simulink subsystem "SiEngineCoreNA"  (R2023b)
settings: Solver=VariableStepAuto  StartTime=0.0  StopTime=10.0  RelTol=1e-3
undefined symbols (not defined in the file): EnvAbsPrs, EnvAirTemp, EnvCpAir, EnvRair, PlntEngCEng, PlntEngCpExh, PlntEngEgrArea, PlntEngExhSysVol, PlntEngGasLhv, PlntEngRexh, PlntEngTauCool, PlntEngTCoolInit, PlntEngTCoolMax, PlntEngTCoolStart, PlntEngThrAngToC, PlntEngVexh, ThrAngToC
libraries: autolibfundflw x10, autolibfundflwcommon x2, simulink x1, autolibpowerinfoutils x1, autolibcoreeng x1
settings Model: ModifiedByFormat=The MathWorks, Inc.  Creator=The MathWorks, Inc.  LastModifiedBy=The MathWorks, Inc.
settings SolverCC: MaxZcPerStep=1
settings OptimizationCC: ReuseModelBlockBuffer=off
settings DebuggingCC: UnconnectedInputMsg=warning  UnconnectedOutputMsg=warning  UnconnectedLineMsg=warning
settings ModelReferenceCC: EnableRefExpFcnMdlSchedulingChecks=on
settings RTWCC: DLArmComputeVersion=19.05

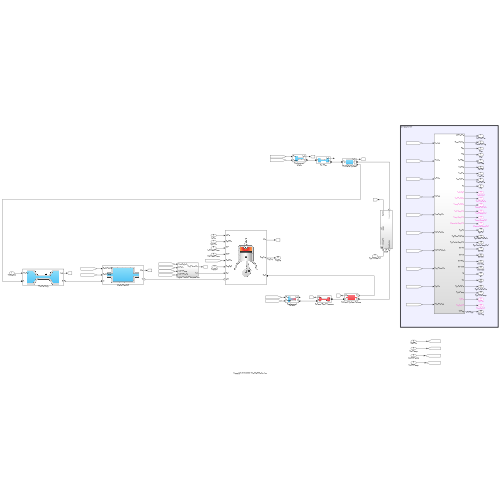
[thumbnail: Simulink's stored preview of the top-level diagram]
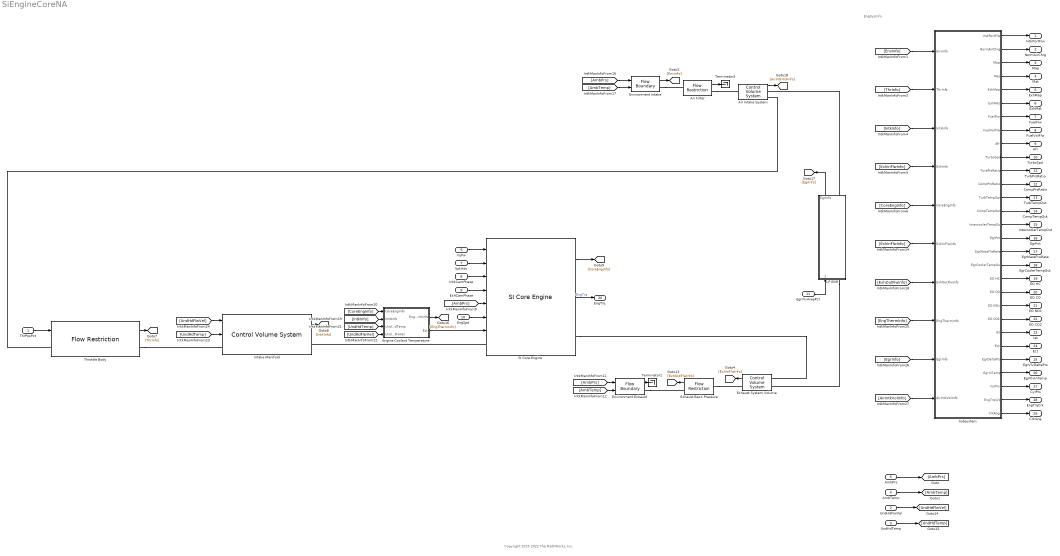
== system SiEngineCoreNA ==
  note: EngSysInfo
  note: Copyright 2015-2022 The MathWorks, Inc.
  ThrPosPct : Inport
  UndHdFlwVel : Inport  Port=2
  UndHdTemp : Inport  Port=3
  AmbTemp : Inport  Port=4
  AmbPrs : Inport  Port=5
  InjPw : Inport  Port=6
  SpkAdv : Inport  Port=7
  IntkCamPhase : Inport  Port=8
  ExhCamPhase : Inport  Port=9
  EngSpd : Inport  Port=10
  EgrVlvAreaPct : Inport  Port=11
  Air Filter : autolibfundflw/Flow Restriction  AreaPopup=Constant  ImageTypePopup=Cold  gamma=EnvCpAir/(EnvCpAir-EnvRair)  R=EnvRair  Plim=0.99  Aorf_cnst=PlntEngAFArea  Cd_cnst=1  Cd_ext=1  Dthr=50  ThrCd=[0.001; 0.735]  ThrAngBpts=[0; 90]
  Air Intake System : autolibfundflw/Control Volume System  NumInletPorts=1  NumOutletPorts=2  HeatTransferModelPopup=Constant  ImageTypePopup=Cold  Vch=PlntEngIntkVol  Pinit=EnvAbsPrs  Tinit=EnvAirTemp  R=EnvRair  cp=EnvCpAir  q_he=0  ext_tbl=[40 160 740 2000]  ext_bpts=linspace(0,180,4)  Aext_conv=0.125  m_wall=7  cp_wall=900  Tmass=293.15  Dext_cond=0.004  Aext_cond=0.003  kext=25  Dint_cond=0.004  Aint_cond=0.003  kint=25  int_tbl=[40 160 740 2000]  int_bpts=linspace(0.0020,0.1100,4)  Aint_conv=0.125
  Engine Coolant Temperature : Subsystem
  Environment Exhaust : autolibfundflw/Flow Boundary  PrsTempSrcPopup=External input  ImageTypePopup=Hot  Pcnst=101325  Tcnst=298.15  cp=EnvCpAir
  Environment Intake : autolibfundflw/Flow Boundary  PrsTempSrcPopup=External input  ImageTypePopup=Cold  Pcnst=101325  Tcnst=298.15  cp=EnvCpAir
  Exhaust Back Pressure : autolibfundflw/Flow Restriction  AreaPopup=Constant  ImageTypePopup=Hot  gamma=PlntEngCpExh/(PlntEngCpExh-PlntEngRexh)  R=PlntEngRexh  Plim=0.99  Aorf_cnst=PlntEngExhSysArea  Cd_cnst=1  Cd_ext=1  Dthr=50  ThrCd=[0.001; 0.735]  ThrAngBpts=[0; 90]
  Exhaust System Volume : autolibfundflw/Control Volume System  NumInletPorts=2  NumOutletPorts=1  HeatTransferModelPopup=Constant  ImageTypePopup=Hot  Vch=PlntEngExhSysVol+PlntEngVexh  Pinit=101325  Tinit=298  R=PlntEngRexh  cp=PlntEngCpExh  q_he=0  ext_tbl=[40 160 740 2000]  ext_bpts=linspace(0,180,4)  Aext_conv=0.125  m_wall=7  cp_wall=900  Tmass=293.15  Dext_cond=0.004  Aext_cond=0.003  kext=25  Dint_cond=0.004  Aint_cond=0.003  kint=25  int_tbl=[40 160 740 2000]  int_bpts=linspace(0.0020,0.1100,4)  Aint_conv=0.125
  Intake Manifold : autolibfundflw/Control Volume System  NumInletPorts=1  NumOutletPorts=1  HeatTransferModelPopup=External wall convection  ImageTypePopup=Cold  Vch=PlntEngVint  Pinit=101325  Tinit=298  R=EnvRair  cp=EnvCpAir  q_he=0  ext_tbl=[40 160 740 2000]  ext_bpts=linspace(0,180,4)  Aext_conv=0.125  m_wall=7  cp_wall=900  Tmass=293.15  Dext_cond=0.004  Aext_cond=0.003  kext=25  Dint_cond=0.004  Aint_cond=0.003  kint=25  int_tbl=[40 160 740 2000]  int_bpts=linspace(0.0020,0.1100,4)  Aint_conv=0.125
  LP EGR : Subsystem  Variant=on  VariantControlMode=label  VariantControl=Choice  LabelModeActiveChoice=LpEGR
  SI Core Engine : autolibcoreeng/SI Core Engine  AirMassFlowOptionPopup=Dual-Independent Variable Cam Phasing  TrqOptionPopup=Torque Structure  NCyl=PlntEngNCyl  Cps=PlntEngCps  Vd=PlntEngVd  Rair=EnvRair  Pstd=EnvAbsPrs  Tstd=EnvAirTemp  f_nv=PlntEngNv  f_nv_prs_bpt=PlntEngNvPrBpt  f_nv_n_bpt=PlntEngNvSpdBpt  f_vivc=PlntEngVivc  f_vivc_icp_bpt=PlntEngVivcBpt  f_tm_corr=PlntEngTmCorr  f_tm_corr_nd_bpt=PlntEngTmCorrNdBpt  f_tm_corr_n_bpt=PlntEngTmCorrNBpt  f_mdot_intk=PlntEngNAMdotIntk  f_mdot_intk_ecp_bpt=PlntEngMdotIntkEcpBpt  f_mdot_trpd_bpt=PlntEngMdotTrpdBpt  f_mdot_air_corr=PlntEngMdotAirCorr  f_mdot_air_corr_ld_bpt=PlntEngMdotAirCorrLdBpt  f_mdot_air_n_bpt=PlntEngMdotAirCorrNBpt  EnableCrkSignalsCheckbox=off  f_crk_firing_frac_bpt=[-1 0 1]  f_crk_prs=PlntEngCrkPrs  f_crk_btq=PlntEngCrkBtq  f_crk_n_bpt=PlntEngCrkNBpt  f_crk_l_bpt=PlntEngCrkLBpt  f_crk_ang_bpt=PlntEngCrkAngBpt  f_crk_tdc_ang=PlntEngCrkTdcAng  f_tq_nl=PlntEngTqTbl  f_tq_nl_l_bpt=PlntEngTqTblLBpt  f_tq_nl_n_bpt=PlntEngTqTblNBpt  f_tq_inr=PlntEngInTrqMapNA  f_tq_fric=PlntEngTqFricNA  f_fric_temp_mod=PlntEngFricTMod  f_fric_temp_bpt=PlntEngFricTBpt  f_tq_pump=PlntEngTqPumpNA  f_sa_opt=PlntEngSAOptNA  f_tq_inr_l_bpt=PlntEngInTrqLdBptNA  f_tq_inr_n_bpt=PlntEngInTrqSpdBptNA  f_m_sa=PlntEngMSa  f_del_sa_bpt=PlntEngDelSaBpt  f_m_lam=PlntEngMLam  f_m_lam_bpt=PlntEngMLamBpt  f_t_exh=PlntEngTexh  f_t_exh_l_bpt=PlntEngTexhLBpt  f_t_exh_n_bpt=PlntEngTexhNBpt  cp_exh=PlntEngCpExh  CO2EmissionsCheckbox=on  COEmissionsCheckbox=on  NOxEmissionsCheckbox=on  HCEmissionsCheckbox=on  PMEmissionsCheckbox=off  f_CO2_frac=PlntEngCO2Frac  f_CO_frac=PlntEngCOFrac  f_HC_frac=PlntEngHCFrac  f_NOx_frac=PlntEngNOxFrac  f_PM_frac=[0 0 0 0 0 0 0 0 0 0 0 0 0 0 0;0 0 0 0 0 0 0 0 0 0 0 0 0 0 0;0 0 0 0 0 0 0 0 0 0 0 0 0 0 0;0 0 0 0 0 0 0 0 0 0 0 0 0 0 0;0 0 0 0 0 0 0 0 0 0 0 0 0 0 0;0 0 0 0 0 0 0 0 0 0 0 0 0 0 0;0 0 0 0 0 0 0 0 0 0 0 0 0 0 0;0 0 0 0 0 0 0 0 0 0 0 0 0 0 0;0 0 0 0 0 0 0 0 0 0 0 0 0 0 0;0 0 0 0 0 0 0 0 0 0 0 0 0 0 0;0 0 0 0 0 0 0 0 0 0 0 0 0 0 0;0 0 0 0 0 0 0 0 0 0 0 0 0 0 0;0 0 0 0 0 0 0 0 0 0 0 0 0 0 0;0 0 0 0 0 0 0 0 0 0 0 0 0 0 0;0 0 0 0 0 0 0 0 0 0 0 0 0 0 0;0 0 0 0 0 0 0 0 0 0 0 0 0 0 0]  f_exhfrac_n_bpt=PlntEngExhFracNBpt  f_exhfrac_trq_bpt=PlntEngExhFracTqBpt  Sinj=PlntEngSinj  afr_stoich=PlntEngAfrStoich  fuel_lhv=PlntEngGasLhv  fuel_sg=PlntEngGasSg
  Subsystem : Subsystem
  Terminator1 : Terminator
  Terminator5 : Terminator
  Throttle Body : autolibfundflw/Flow Restriction  AreaPopup=Throttle body geometry  ImageTypePopup=Cold  gamma=EnvCpAir / (EnvCpAir - EnvRair)  R=EnvRair  Plim=0.99  Aorf_cnst=.1  Cd_cnst=1  Cd_ext=1  Dthr=PlntEngThrDia  ThrCd=PlntEngThrAngToC(:,2)  ThrAngBpts=PlntEngThrAngToC(:,1)
  IntkPortFlw : Outport  VectorParamsAs1DForOutWhenUnconnected=off
  NormAirChrg : Outport  Port=2  VectorParamsAs1DForOutWhenUnconnected=off
  Map : Outport  Port=3  VectorParamsAs1DForOutWhenUnconnected=off
  Mat : Outport  Port=4  VectorParamsAs1DForOutWhenUnconnected=off
  ExhMap : Outport  Port=5  VectorParamsAs1DForOutWhenUnconnected=off
  ExhMat : Outport  Port=6  VectorParamsAs1DForOutWhenUnconnected=off
  FuelFlw : Outport  Port=7  VectorParamsAs1DForOutWhenUnconnected=off
  FuelVolFlw : Outport  Port=8  VectorParamsAs1DForOutWhenUnconnected=off
  Afr : Outport  Port=9  VectorParamsAs1DForOutWhenUnconnected=off
  TurboSpd : Outport  Port=10  VectorParamsAs1DForOutWhenUnconnected=off
  TurbPrsRatio : Outport  Port=11  VectorParamsAs1DForOutWhenUnconnected=off
  CompPrsRatio : Outport  Port=12  VectorParamsAs1DForOutWhenUnconnected=off
  TurbTempOut : Outport  Port=13  VectorParamsAs1DForOutWhenUnconnected=off
  CompTempOut : Outport  Port=14  VectorParamsAs1DForOutWhenUnconnected=off
  IntercoolerTempOut : Outport  Port=15  VectorParamsAs1DForOutWhenUnconnected=off
  EgrPct : Outport  Port=16  VectorParamsAs1DForOutWhenUnconnected=off
  EgrMassFlwRate : Outport  Port=17  VectorParamsAs1DForOutWhenUnconnected=off
  EgrCoolerTempOut : Outport  Port=18  VectorParamsAs1DForOutWhenUnconnected=off
  EO HC : Outport  Port=19  VectorParamsAs1DForOutWhenUnconnected=off
  EO CO : Outport  Port=20  VectorParamsAs1DForOutWhenUnconnected=off
  EO NOx : Outport  Port=21  VectorParamsAs1DForOutWhenUnconnected=off
  EO CO2 : Outport  Port=22  VectorParamsAs1DForOutWhenUnconnected=off
  Iat : Outport  Port=23  VectorParamsAs1DForOutWhenUnconnected=off
  Ect : Outport  Port=24  VectorParamsAs1DForOutWhenUnconnected=off
  EgrVlvDeltaPrs : Outport  Port=25  VectorParamsAs1DForOutWhenUnconnected=off
  EgrVlvInTemp : Outport  Port=26  VectorParamsAs1DForOutWhenUnconnected=off
  CylPrs : Outport  Port=27  VectorParamsAs1DForOutWhenUnconnected=off
  EngTrqCrk : Outport  Port=28  VectorParamsAs1DForOutWhenUnconnected=off
  CrkAng : Outport  Port=29  VectorParamsAs1DForOutWhenUnconnected=off
  EngTrq : Outport  Port=30  VectorParamsAs1DForOutWhenUnconnected=off
  wires:
  [ExhInFlwInfo] -> Subsystem/4(ExhInfo)
  Subsystem/14(CompTempOut) -> CompTempOut/1
  Subsystem/29(CrkAng) -> CrkAng/1
  Subsystem/28(EngTrqCrk) -> EngTrqCrk/1
  Subsystem/12(CompPrsRatio) -> CompPrsRatio/1
  Subsystem/6(ExhMat) -> ExhMat/1
  Subsystem/8(FuelVolFlw) -> FuelVolFlw/1
  AmbTemp/1 -> [AmbTemp]
  Subsystem/13(TurbTempOut) -> TurbTempOut/1
  Subsystem/27(CylPrs) -> CylPrs/1
  Subsystem/15(IntercoolerTempOut) -> IntercoolerTempOut/1
  [UndHdFlwVel] -> Intake Manifold/1
  Subsystem/24(Ect) -> Ect/1
  Subsystem/11(TurbPrsRatio) -> TurbPrsRatio/1
  Subsystem/23(Iat) -> Iat/1
  Subsystem/10(TurboSpd) -> TurboSpd/1
  AmbPrs/1 -> [AmbPrs]
  Subsystem/22(EO CO2) -> EO CO2/1
  Subsystem/3(Map) -> Map/1
  Subsystem/9(Afr) -> Afr/1
  Subsystem/25(EgrDeltaPrs) -> EgrVlvDeltaPrs/1
  Subsystem/26(EgrInTemp) -> EgrVlvInTemp/1
  Subsystem/21(EO NOx) -> EO NOx/1
  Subsystem/4(Mat) -> Mat/1
  Subsystem/5(ExhMap) -> ExhMap/1
  [AirIntkVolInfo] -> Subsystem/10(AirIntkVolInfo)
  [AmbPrs] -> Environment Intake/1
  Subsystem/16(EgrPct) -> EgrPct/1
  [CoreEngInfo] -> Subsystem/5(CoreEngInfo)
  Subsystem/20(EO CO) -> EO CO/1
  Subsystem/7(FuelFlw) -> FuelFlw/1
  [EgrInfo] -> Subsystem/9(EgrInfo)
  [ExhOutFlwInfo] -> Subsystem/7(ExhOutFlwInfo)
  [EngThermInfo] -> Subsystem/8(EngThermInfo)
  [ExhInFlwInfo] -> Subsystem/6(ExhInFlwInfo)
  ThrPosPct/1 -> Throttle Body/1
  [UndHdTemp] -> Intake Manifold/2
  UndHdFlwVel/1 -> [UndHdFlwVel]
  UndHdTemp/1 -> [UndHdTemp]
  Intake Manifold/1 -> [IntkInfo]
  Exhaust Back Pressure/1 -> [ExhOutFlwInfo]
  [EnvInfo] -> Subsystem/1(EnvInfo)
  Environment Intake/1 -> [EnvInfo]
  Subsystem/18(EgrCoolerTempOut) -> EgrCoolerTempOut/1
  Exhaust System Volume/1 -> [ExhInFlwInfo]
  Environment Exhaust/1 -> Terminator1/1
  Subsystem/19(EO HC) -> EO HC/1
  [AmbTemp] -> Environment Exhaust/2
  Subsystem/2(NormAirChrg) -> NormAirChrg/1
  Subsystem/1(IntkPortFlw) -> IntkPortFlw/1
  [AmbPrs] -> Environment Exhaust/1
  [AmbTemp] -> Environment Intake/2
  Air Filter/1 -> Terminator5/1
  Throttle Body/1 -> [ThrInfo]
  [IntkInfo] -> Subsystem/3(IntkInfo)
  Subsystem/17(EgrMassFlwRate) -> EgrMassFlwRate/1
  Air Intake System/1 -> [AirIntkVolInfo]
  [ThrInfo] -> Subsystem/2(ThrInfo)
  SpkAdv/1 -> SI Core Engine/2
  ExhCamPhase/1 -> SI Core Engine/4
  IntkCamPhase/1 -> SI Core Engine/3
  EngSpd/1 -> SI Core Engine/6
  SI Core Engine/1 -> [CoreEngInfo]
  InjPw/1 -> SI Core Engine/1
  [UndHdTemp] -> Engine Coolant Temperature/3(UndHdTemp)
  Engine Coolant Temperature/2(Ect) -> SI Core Engine/7
  [IntkInfo] -> Engine Coolant Temperature/2(IntkInfo)
  [CoreEngInfo] -> Engine Coolant Temperature/1(CoreEngInfo)
  [AmbPrs] -> SI Core Engine/5
  [UndHdFlwVel] -> Engine Coolant Temperature/4(UndHdFlwVel)
  SI Core Engine/2 -> EngTrq/1  "EngTrq"
  Engine Coolant Temperature/1(EngThermInfo) -> [EngThermInfo]
  LP EGR/1(EgrInfo) -> [EgrInfo]
  EgrVlvAreaPct/1 -> LP EGR/1(EgrVlvAreaPct)
  connections:
  Throttle Body/LConn1 -- Air Intake System/RConn2
  Air Filter/RConn1 -- Air Intake System/LConn1
  Throttle Body/RConn1 -- Intake Manifold/LConn1
  Environment Intake/RConn1 -- Air Filter/LConn1
  Exhaust Back Pressure/LConn1 -- Exhaust System Volume/RConn1
  Environment Exhaust/RConn1 -- Exhaust Back Pressure/RConn1
  SI Core Engine/RConn1 -- Exhaust System Volume/LConn1
  SI Core Engine/LConn1 -- Intake Manifold/RConn1
  LP EGR/RConn1 -- Air Intake System/RConn1
  LP EGR/LConn1 -- Exhaust System Volume/LConn2

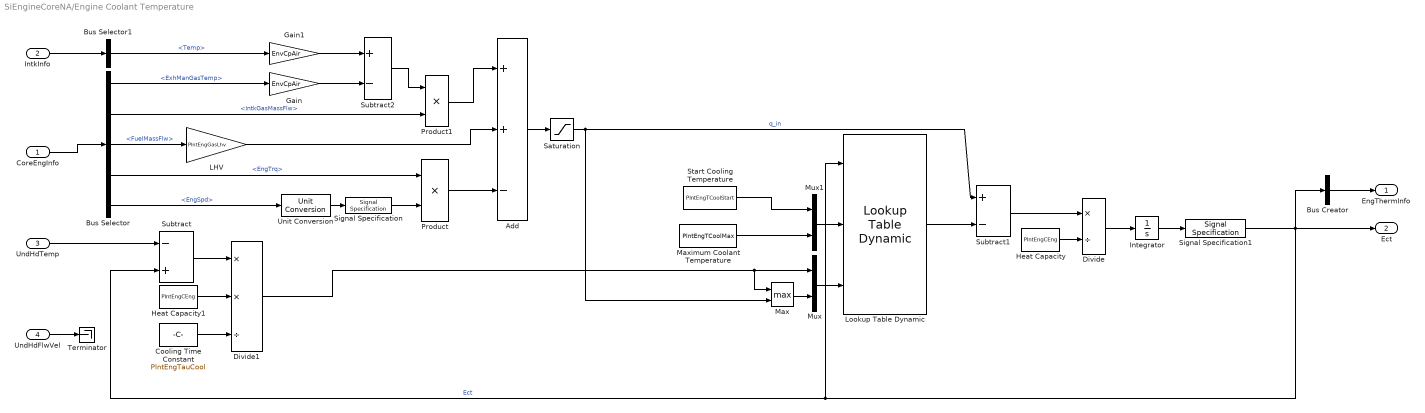
== system SiEngineCoreNA/Engine Coolant Temperature ==
  CoreEngInfo : Inport
  IntkInfo : Inport  Port=2
  UndHdTemp : Inport  Port=3
  UndHdFlwVel : Inport  Port=4
  Add : Sum  Inputs=++-
  Bus Creator : BusCreator  Inputs=1
  Bus Selector : BusSelector  OutputSignals=ExhManGasTemp,IntkGasMassFlw,FuelMassFlw,EngTrq,EngSpd
  Bus Selector1 : BusSelector  OutputSignals=Vol.Temp
  Cooling Time Constant : Constant  Value=PlntEngTauCool
  Divide : Product  Inputs=*/
  Divide1 : Product  Inputs=**/
  Gain : Gain  Gain=EnvCpAir
  Gain1 : Gain  Gain=EnvCpAir
  Heat Capacity : Constant  Value=PlntEngCEng
  Heat Capacity1 : Constant  Value=PlntEngCEng
  Integrator : Integrator  InitialCondition=PlntEngTCoolInit  LimitOutput=on  UpperSaturationLimit=PlntEngTCoolMax  LowerSaturationLimit=0  ZeroCross=off
  LHV : Gain  Gain=PlntEngGasLhv
  Lookup Table Dynamic : simulink/Lookup Tables/Lookup Table Dynamic  LookUpMeth=Interpolation-Use End Values  OutDataType=fixdt('double')  OutScaling=[]  OutputDataTypeScalingMode=Specify via dialog  OutDataTypeStr=double  DoSatur=off
  Max : MinMax  Function=max  Inputs=2  ZeroCross=off
  Maximum Coolant Temperature : Constant  Value=PlntEngTCoolMax
  Mux : Mux  Inputs=2
  Mux1 : Mux  Inputs=2
  Product : Product
  Product1 : Product
  Saturation : Saturate  UpperLimit=Inf  LowerLimit=0
  Signal Specification : SignalSpecification  Unit=rad/s
  Signal Specification1 : SignalSpecification  Unit=K
  Start Cooling Temperature : Constant  Value=PlntEngTCoolStart
  Subtract : Sum  Inputs=-+
  Subtract1 : Sum  Inputs=+-
  Subtract2 : Sum  Inputs=+-
  Terminator : Terminator
  Unit Conversion : UnitConversion
  EngThermInfo : Outport  Unit=K  VectorParamsAs1DForOutWhenUnconnected=off
  Ect : Outport  Port=2  Unit=K  VectorParamsAs1DForOutWhenUnconnected=off
  wires:
  Add/1 -> Saturation/1
  Product1/1 -> Add/1
  Bus Selector/2 -> Product1/2  "<IntkGasMassFlw>"
  Subtract2/1 -> Product1/1
  Integrator/1 -> Signal Specification1/1
  IntkInfo/1 -> Bus Selector1/1
  Bus Creator/1 -> EngThermInfo/1
  Max/1 -> Mux/2
  Lookup Table Dynamic/1 -> Subtract1/2
  Subtract1/1 -> Divide/1
  Divide/1 -> Integrator/1
  Bus Selector1/1 -> Gain1/1  "<Temp>"
  Gain1/1 -> Subtract2/1
  Bus Selector/1 -> Gain/1  "<ExhManGasTemp>"
  Bus Selector/3 -> LHV/1  "<FuelMassFlw>"
  CoreEngInfo/1 -> Bus Selector/1
  Cooling Time Constant/1 -> Divide1/3
  Bus Selector/5 -> Unit Conversion/1  "<EngSpd>"
  Product/1 -> Add/3
  LHV/1 -> Add/2
  Signal Specification/1 -> Product/2
  Saturation/1 -> Subtract1/1, Max/2  "q_in"
  Subtract/1 -> Divide1/1
  Start Cooling Temperature/1 -> Mux1/1
  Mux/1 -> Lookup Table Dynamic/3
  Heat Capacity1/1 -> Divide1/2
  Divide1/1 -> Mux/1, Max/1
  Mux1/1 -> Lookup Table Dynamic/2
  Bus Selector/4 -> Product/1  "<EngTrq>"
  Gain/1 -> Subtract2/2
  UndHdFlwVel/1 -> Terminator/1
  Signal Specification1/1 -> Ect/1, Bus Creator/1, Lookup Table Dynamic/1, Subtract/2  "Ect"
  Maximum Coolant Temperature/1 -> Mux1/2
  Unit Conversion/1 -> Signal Specification/1
  Heat Capacity/1 -> Divide/2
  UndHdTemp/1 -> Subtract/1

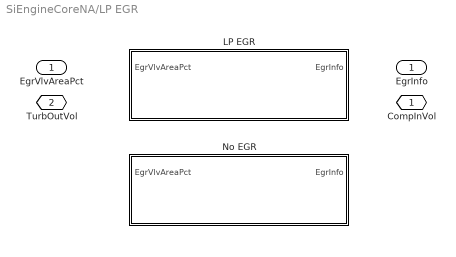
== system SiEngineCoreNA/LP EGR ==
  EgrVlvAreaPct : Inport
  LP EGR : Subsystem  VariantControl=LpEGR
  No EGR : Subsystem  VariantControl=NoEGR
  CompInVol : PMIOPort  Side=Right
  TurbOutVol : PMIOPort  Port=2  Side=Left
  EgrInfo : Outport

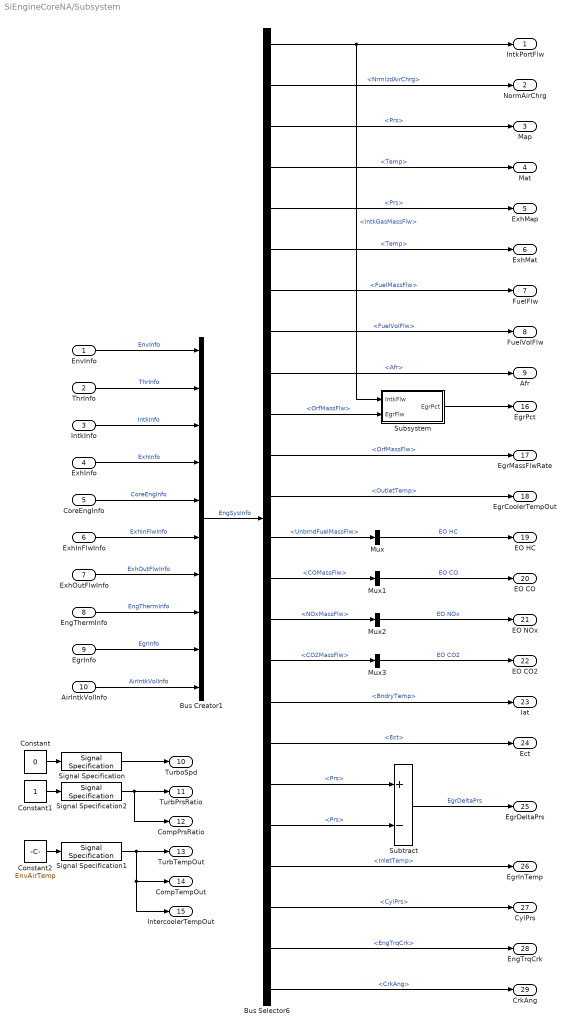
== system SiEngineCoreNA/Subsystem ==
  EnvInfo : Inport
  ThrInfo : Inport  Port=2
  IntkInfo : Inport  Port=3
  ExhInfo : Inport  Port=4
  CoreEngInfo : Inport  Port=5
  ExhInFlwInfo : Inport  Port=6
  ExhOutFlwInfo : Inport  Port=7
  EngThermInfo : Inport  Port=8
  EgrInfo : Inport  Port=9
  AirIntkVolInfo : Inport  Port=10
  Bus Creator1 : BusCreator  Inputs=10
  Bus Selector6 : BusSelector  OutputSignals=CoreEngInfo.IntkGasMassFlw,CoreEngInfo.NrmlzdAirChrg,IntkInfo.Vol.Prs,IntkInfo.Vol.Temp,ExhInfo.Vol.Prs,ExhInfo.Vol.Temp,CoreEngInfo.FuelMassFlw,CoreEngInfo.FuelVolFlw,CoreEngInfo.Afr,EgrInfo.EgrVlv.Flw.OrfMassFlw,EgrInfo.EgrVlv.Flw.OrfMassFlw,EgrInfo.EgrCooler.OutletTemp,ExhOutFlwInfo.Flw.Species.UnbrndFuelMassFlw,ExhOutFlwInfo.Flw.Species.COMassFlw,ExhOutFlwInfo.Flw.Species.NOxMassFlw,ExhOutFlwInfo.Flw.Species.CO2MassFlw,EnvInfo.BndryTemp,EngThermInfo.Ect,ExhInFlwInfo.Vol.Prs,AirIntkVolInfo.Vol.Prs,EgrInfo.EgrCooler.InletTemp,CoreEngInfo.CylPrs,CoreEngInfo.EngTrqCrk,CoreEngInfo.CrkAng
  Constant : Constant  Value=0
  Constant1 : Constant
  Constant2 : Constant  Value=EnvAirTemp
  Mux{,1..3} (4 alike) : Mux  Inputs=1
  Signal Specification : SignalSpecification  Unit=rad/sec
  Signal Specification1 : SignalSpecification  Unit=K
  Signal Specification2 : SignalSpecification  Unit=1
  Subsystem : Subsystem
  Subtract : Sum  Inputs=+-
  IntkPortFlw : Outport  VectorParamsAs1DForOutWhenUnconnected=off
  NormAirChrg : Outport  Port=2  Unit=1  VectorParamsAs1DForOutWhenUnconnected=off
  Map : Outport  Port=3  VectorParamsAs1DForOutWhenUnconnected=off
  Mat : Outport  Port=4  VectorParamsAs1DForOutWhenUnconnected=off
  ExhMap : Outport  Port=5  VectorParamsAs1DForOutWhenUnconnected=off
  ExhMat : Outport  Port=6  VectorParamsAs1DForOutWhenUnconnected=off
  FuelFlw : Outport  Port=7  VectorParamsAs1DForOutWhenUnconnected=off
  FuelVolFlw : Outport  Port=8  VectorParamsAs1DForOutWhenUnconnected=off
  Afr : Outport  Port=9  Unit=1  VectorParamsAs1DForOutWhenUnconnected=off
  TurboSpd : Outport  Port=10  VectorParamsAs1DForOutWhenUnconnected=off
  TurbPrsRatio : Outport  Port=11  VectorParamsAs1DForOutWhenUnconnected=off
  CompPrsRatio : Outport  Port=12  VectorParamsAs1DForOutWhenUnconnected=off
  TurbTempOut : Outport  Port=13  VectorParamsAs1DForOutWhenUnconnected=off
  CompTempOut : Outport  Port=14  VectorParamsAs1DForOutWhenUnconnected=off
  IntercoolerTempOut : Outport  Port=15  VectorParamsAs1DForOutWhenUnconnected=off
  EgrPct : Outport  Port=16  Unit=%  VectorParamsAs1DForOutWhenUnconnected=off
  EgrMassFlwRate : Outport  Port=17  VectorParamsAs1DForOutWhenUnconnected=off
  EgrCoolerTempOut : Outport  Port=18  VectorParamsAs1DForOutWhenUnconnected=off
  EO HC : Outport  Port=19  VectorParamsAs1DForOutWhenUnconnected=off
  EO CO : Outport  Port=20  VectorParamsAs1DForOutWhenUnconnected=off
  EO NOx : Outport  Port=21  VectorParamsAs1DForOutWhenUnconnected=off
  EO CO2 : Outport  Port=22  VectorParamsAs1DForOutWhenUnconnected=off
  Iat : Outport  Port=23  VectorParamsAs1DForOutWhenUnconnected=off
  Ect : Outport  Port=24  VectorParamsAs1DForOutWhenUnconnected=off
  EgrDeltaPrs : Outport  Port=25  Unit=Pa  VectorParamsAs1DForOutWhenUnconnected=off
  EgrInTemp : Outport  Port=26  Unit=K  VectorParamsAs1DForOutWhenUnconnected=off
  CylPrs : Outport  Port=27  VectorParamsAs1DForOutWhenUnconnected=off
  EngTrqCrk : Outport  Port=28  VectorParamsAs1DForOutWhenUnconnected=off
  CrkAng : Outport  Port=29  VectorParamsAs1DForOutWhenUnconnected=off
  wires:
  IntkInfo/1 -> Bus Creator1/3  "IntkInfo"
  ExhInfo/1 -> Bus Creator1/4  "ExhInfo"
  CoreEngInfo/1 -> Bus Creator1/5  "CoreEngInfo"
  EnvInfo/1 -> Bus Creator1/1  "EnvInfo"
  Bus Creator1/1 -> Bus Selector6/1  "EngSysInfo"
  ThrInfo/1 -> Bus Creator1/2  "ThrInfo"
  Bus Selector6/1 -> Subsystem/1(IntkFlw), IntkPortFlw/1  "<IntkGasMassFlw>"
  Bus Selector6/3 -> Map/1  "<Prs>"
  Bus Selector6/4 -> Mat/1  "<Temp>"
  Bus Selector6/5 -> ExhMap/1  "<Prs>"
  Bus Selector6/6 -> ExhMat/1  "<Temp>"
  Bus Selector6/7 -> FuelFlw/1  "<FuelMassFlw>"
  Bus Selector6/9 -> Afr/1  "<Afr>"
  Bus Selector6/2 -> NormAirChrg/1  "<NrmlzdAirChrg>"
  Mux/1 -> EO HC/1  "EO HC"
  Mux2/1 -> EO NOx/1  "EO NOx"
  Mux3/1 -> EO CO2/1  "EO CO2"
  Mux1/1 -> EO CO/1  "EO CO"
  Bus Selector6/13 -> Mux/1  "<UnbrndFuelMassFlw>"
  Bus Selector6/14 -> Mux1/1  "<COMassFlw>"
  Bus Selector6/15 -> Mux2/1  "<NOxMassFlw>"
  Bus Selector6/16 -> Mux3/1  "<CO2MassFlw>"
  Bus Selector6/18 -> Ect/1  "<Ect>"
  Bus Selector6/12 -> EgrCoolerTempOut/1  "<OutletTemp>"
  Subsystem/1(EgrPct) -> EgrPct/1
  Bus Selector6/20 -> Subtract/2  "<Prs>"
  Subtract/1 -> EgrDeltaPrs/1  "EgrDeltaPrs"
  Bus Selector6/21 -> EgrInTemp/1  "<InletTemp>"
  Bus Selector6/11 -> EgrMassFlwRate/1  "<OrfMassFlw>"
  Bus Selector6/10 -> Subsystem/2(EgrFlw)  "<OrfMassFlw>"
  Bus Selector6/17 -> Iat/1  "<BndryTemp>"
  Bus Selector6/8 -> FuelVolFlw/1  "<FuelVolFlw>"
  AirIntkVolInfo/1 -> Bus Creator1/10  "AirIntkVolInfo"
  EgrInfo/1 -> Bus Creator1/9  "EgrInfo"
  EngThermInfo/1 -> Bus Creator1/8  "EngThermInfo"
  ExhOutFlwInfo/1 -> Bus Creator1/7  "ExhOutFlwInfo"
  ExhInFlwInfo/1 -> Bus Creator1/6  "ExhInFlwInfo"
  Bus Selector6/19 -> Subtract/1  "<Prs>"
  Constant/1 -> Signal Specification/1
  Constant1/1 -> Signal Specification2/1
  Constant2/1 -> Signal Specification1/1
  Signal Specification/1 -> TurboSpd/1
  Signal Specification1/1 -> IntercoolerTempOut/1, CompTempOut/1, TurbTempOut/1
  Signal Specification2/1 -> CompPrsRatio/1, TurbPrsRatio/1
  Bus Selector6/22 -> CylPrs/1  "<CylPrs>"
  Bus Selector6/23 -> EngTrqCrk/1  "<EngTrqCrk>"
  Bus Selector6/24 -> CrkAng/1  "<CrkAng>"

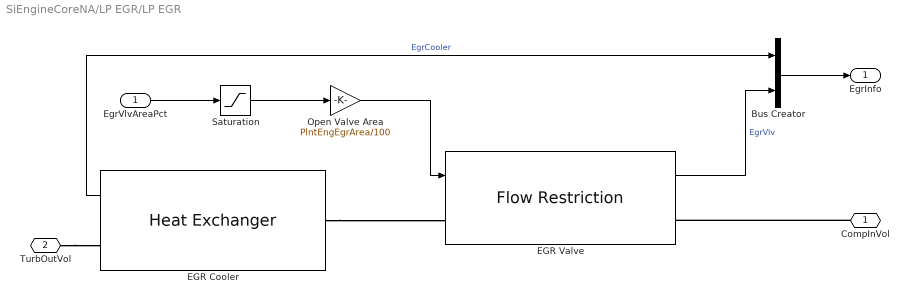
== system SiEngineCoreNA/LP EGR/LP EGR ==
  EgrVlvAreaPct : Inport
  Bus Creator : BusCreator  Inputs=2
  EGR Cooler : autolibfundflw/Heat Exchanger  EffctModelPopup=Constant  CoolTempInputPopup=Constant  ImageTypePopup=EGR cooler cold to hot  ep_cnst=PlntEngEgrEff  T_cool_cnst=PlntEngEgrEff  cp=PlntEngCpExh
  EGR Valve : autolibfundflw/Flow Restriction  AreaPopup=External input  ImageTypePopup=Cold  gamma=PlntEngCpExh / (PlntEngCpExh - PlntEngRexh)  R=EnvRair  Plim=0.99  Aorf_cnst=.1  Cd_cnst=1  Cd_ext=1  Dthr=ThrDiam  ThrCd=ThrAngToC(:,2)  ThrAngBpts=ThrAngToC(:,1)
  Open Valve Area : Gain  Gain=PlntEngEgrArea/100
  Saturation : Saturate  UpperLimit=100  LowerLimit=0
  CompInVol : PMIOPort  Side=Right
  TurbOutVol : PMIOPort  Port=2  Side=Left
  EgrInfo : Outport  VectorParamsAs1DForOutWhenUnconnected=off
  wires:
  EGR Valve/1 -> Bus Creator/2  "EgrVlv"
  EGR Cooler/1 -> Bus Creator/1  "EgrCooler"
  Bus Creator/1 -> EgrInfo/1
  Saturation/1 -> Open Valve Area/1
  Open Valve Area/1 -> EGR Valve/1
  EgrVlvAreaPct/1 -> Saturation/1
  connections:
  CompInVol/RConn1 -- EGR Valve/RConn1
  EGR Cooler/LConn1 -- EGR Valve/LConn1
  TurbOutVol/RConn1 -- EGR Cooler/RConn1

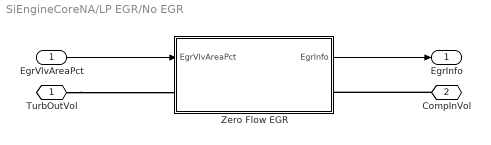
== system SiEngineCoreNA/LP EGR/No EGR ==
  EgrVlvAreaPct : Inport
  Zero Flow EGR : Subsystem
  TurbOutVol : PMIOPort  Side=Left
  CompInVol : PMIOPort  Port=2  Side=Right
  EgrInfo : Outport  VectorParamsAs1DForOutWhenUnconnected=off
  wires:
  Zero Flow EGR/1(EgrInfo) -> EgrInfo/1
  EgrVlvAreaPct/1 -> Zero Flow EGR/1(EgrVlvAreaPct)
  connections:
  TurbOutVol/RConn1 -- Zero Flow EGR/LConn1
  CompInVol/RConn1 -- Zero Flow EGR/RConn1

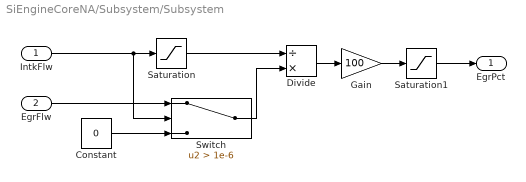
== system SiEngineCoreNA/Subsystem/Subsystem ==
  IntkFlw : Inport
  EgrFlw : Inport  Port=2
  Constant : Constant  Value=0
  Divide : Product  Inputs=/*
  Gain : Gain  Gain=100
  Saturation : Saturate  UpperLimit=1e6  LowerLimit=1e-6  ZeroCross=off
  Saturation1 : Saturate  UpperLimit=100  LowerLimit=0  ZeroCross=off
  Switch : Switch  Criteria=u2 > Threshold  Threshold=1e-6  ZeroCross=off  SaturateOnIntegerOverflow=off  InputSameDT=off
  EgrPct : Outport  VectorParamsAs1DForOutWhenUnconnected=off
  wires:
  Constant/1 -> Switch/3
  Divide/1 -> Gain/1
  Switch/1 -> Divide/2
  Saturation/1 -> Divide/1
  Gain/1 -> Saturation1/1
  EgrFlw/1 -> Switch/1
  IntkFlw/1 -> Switch/2, Saturation/1
  Saturation1/1 -> EgrPct/1

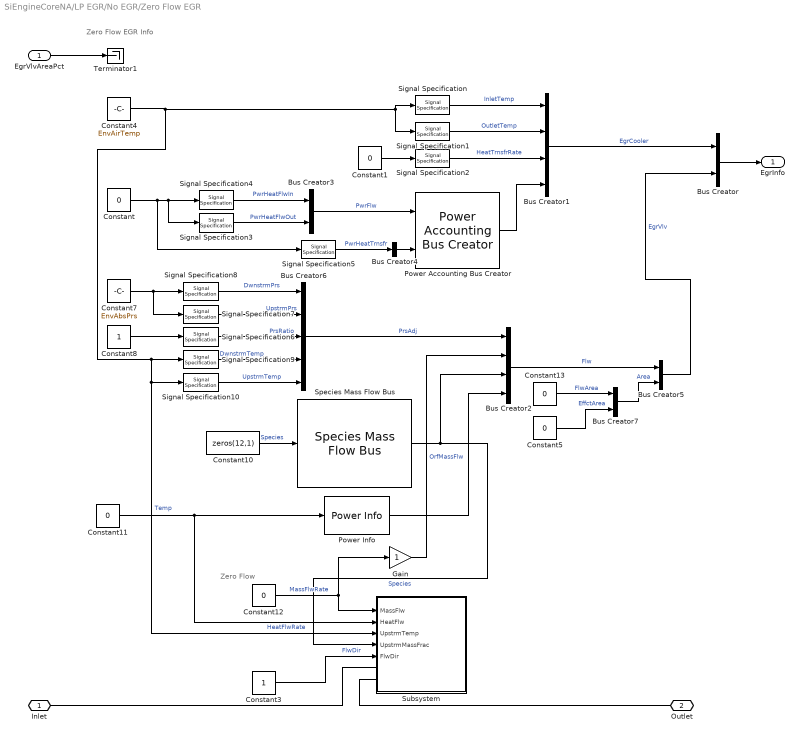
== system SiEngineCoreNA/LP EGR/No EGR/Zero Flow EGR ==
  note: Zero Flow
  note: Zero Flow EGR Info
  EgrVlvAreaPct : Inport
  Bus Creator{,3,5,7} (4 alike) : BusCreator  Inputs=2
  Bus Creator1 : BusCreator  Inputs=4
  Bus Creator2 : BusCreator  Inputs=4
  Bus Creator4 : BusCreator  Inputs=1
  Bus Creator6 : BusCreator  Inputs=5
  Constant{,1,5,11..13} (6 alike) : Constant  Value=0
  Constant10 : Constant  Value=zeros(12,1)
  Constant3 : Constant
  Constant4 : Constant  Value=EnvAirTemp
  Constant7 : Constant  Value=EnvAbsPrs
  Constant8 : Constant
  Gain : Gain
  Power Accounting Bus Creator : autolibpowerinfoutils/Power Accounting Bus Creator  AssctBlkSelPopup=Parent reference block  RefBlkName='autolibfundflw/Heat Exchanger'  PwrTrnsfrdCheckBox=on  PwrNotTrnsfrdCheckBox=on  PwrStoredCheckBox=off  aMode=aMode
  Power Info : autolibfundflwcommon/Compressible Flow Orifice/Power Info  SystemSampleTime=-1  VariantActivationTime=update diagram  AllowFlexibleInterface=on  Latency=0  AutoFrameSizeCalculation=off
  Signal Specification{,1,9..10} (4 alike) : SignalSpecification  Unit=K
  Signal Specification2 : SignalSpecification  Unit=J/s
  Signal Specification3 : SignalSpecification  Unit=W
  Signal Specification4 : SignalSpecification  Unit=W
  Signal Specification5 : SignalSpecification  Unit=W
  Signal Specification6 : SignalSpecification  Unit=1
  Signal Specification7 : SignalSpecification  Unit=Pa
  Signal Specification8 : SignalSpecification  Unit=Pa
  Species Mass Flow Bus : autolibfundflwcommon/Species Mass Flow Bus  SystemSampleTime=-1  VariantActivationTime=update diagram  AllowFlexibleInterface=on  Latency=0  AutoFrameSizeCalculation=off
  Subsystem : Subsystem
  Terminator1 : Terminator
  Inlet : PMIOPort  Side=Right
  Outlet : PMIOPort  Port=2  Side=Left
  EgrInfo : Outport  VectorParamsAs1DForOutWhenUnconnected=off
  wires:
  Signal Specification4/1 -> Bus Creator3/1  "PwrHeatFlwIn"
  Bus Creator3/1 -> Power Accounting Bus Creator/1  "PwrFlw"
  Signal Specification5/1 -> Bus Creator4/1  "PwrHeatTrnsfr"
  Power Accounting Bus Creator/1 -> Bus Creator1/4
  Gain/1 -> Bus Creator2/2  "OrfMassFlw"
  Signal Specification6/1 -> Bus Creator6/3  "PrsRatio"
  Signal Specification1/1 -> Bus Creator1/2  "OutletTemp"
  Bus Creator5/1 -> Bus Creator/2  "EgrVlv"
  Bus Creator7/1 -> Bus Creator5/2  "Area"
  Signal Specification2/1 -> Bus Creator1/3  "HeatTrnsfrRate"
  Species Mass Flow Bus/1 -> Subsystem/4(UpstrmMassFrac), Bus Creator2/3  "Species"
  Signal Specification/1 -> Bus Creator1/1  "InletTemp"
  Power Info/1 -> Bus Creator2/4
  Constant4/1 -> Signal Specification1/1, Signal Specification/1, Signal Specification9/1, Signal Specification10/1, Subsystem/3(UpstrmTemp)  "Temp"
  Constant7/1 -> Signal Specification8/1, Signal Specification7/1
  Bus Creator2/1 -> Bus Creator5/1  "Flw"
  Signal Specification3/1 -> Bus Creator3/2  "PwrHeatFlwOut"
  Constant11/1 -> Power Info/1, Subsystem/2(HeatFlw)  "HeatFlwRate"
  Bus Creator4/1 -> Power Accounting Bus Creator/2
  Bus Creator/1 -> EgrInfo/1
  Constant/1 -> Signal Specification4/1, Signal Specification3/1, Signal Specification5/1
  Constant8/1 -> Signal Specification6/1
  Signal Specification9/1 -> Bus Creator6/4  "DwnstrmTemp"
  Signal Specification7/1 -> Bus Creator6/2  "UpstrmPrs"
  EgrVlvAreaPct/1 -> Terminator1/1
  Constant1/1 -> Signal Specification2/1
  Bus Creator1/1 -> Bus Creator/1  "EgrCooler"
  Constant12/1 -> Subsystem/1(MassFlw), Gain/1  "MassFlwRate"
  Signal Specification10/1 -> Bus Creator6/5  "UpstrmTemp"
  Constant3/1 -> Subsystem/5(FlwDir)  "FlwDir"
  Signal Specification8/1 -> Bus Creator6/1  "DwnstrmPrs"
  Constant10/1 -> Species Mass Flow Bus/1  "Species"
  Constant5/1 -> Bus Creator7/2  "EffctArea"
  Constant13/1 -> Bus Creator7/1  "FlwArea"
  Bus Creator6/1 -> Bus Creator2/1  "PrsAdj"
  connections:
  Subsystem/LConn2 -- Outlet/RConn1
  Subsystem/LConn1 -- Inlet/RConn1

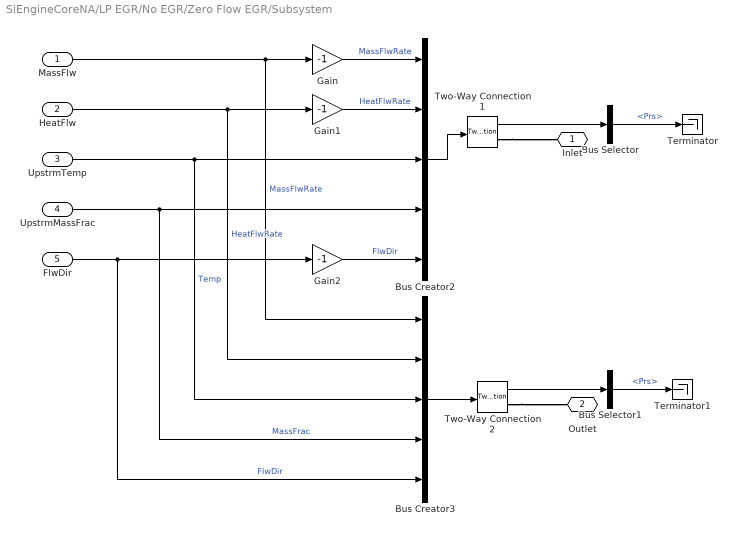
== system SiEngineCoreNA/LP EGR/No EGR/Zero Flow EGR/Subsystem ==
  MassFlw : Inport
  HeatFlw : Inport  Port=2
  UpstrmTemp : Inport  Port=3
  UpstrmMassFrac : Inport  Port=4
  FlwDir : Inport  Port=5
  Bus Creator2 : BusCreator  Inputs=5
  Bus Creator3 : BusCreator  Inputs=5
  Bus Selector : BusSelector  OutputSignals=Prs
  Bus Selector1 : BusSelector  OutputSignals=Prs
  Gain : Gain  Gain=-1
  Gain1 : Gain  Gain=-1
  Gain2 : Gain  Gain=-1
  Terminator : Terminator
  Terminator1 : Terminator
  Two-Way Connection1 : TwoWayConnection
  Two-Way Connection2 : TwoWayConnection
  Inlet : PMIOPort  Side=Left
  Outlet : PMIOPort  Port=2  Side=Left
  wires:
  Gain/1 -> Bus Creator2/1  "MassFlwRate"
  Bus Creator2/1 -> Two-Way Connection1/1
  Gain1/1 -> Bus Creator2/2  "HeatFlwRate"
  Gain2/1 -> Bus Creator2/5  "FlwDir"
  UpstrmMassFrac/1 -> Bus Creator3/4, Bus Creator2/4  "MassFrac"
  HeatFlw/1 -> Gain1/1, Bus Creator3/2  "HeatFlwRate"
  MassFlw/1 -> Bus Creator3/1, Gain/1  "MassFlwRate"
  UpstrmTemp/1 -> Bus Creator2/3, Bus Creator3/3  "Temp"
  Bus Creator3/1 -> Two-Way Connection2/1
  FlwDir/1 -> Bus Creator3/5, Gain2/1  "FlwDir"
  Two-Way Connection1/1 -> Bus Selector/1
  Bus Selector/1 -> Terminator/1  "<Prs>"
  Bus Selector1/1 -> Terminator1/1  "<Prs>"
  Two-Way Connection2/1 -> Bus Selector1/1
  connections:
  Two-Way Connection2/RConn1 -- Outlet/RConn1
  Two-Way Connection1/RConn1 -- Inlet/RConn1
